simulink model "design_sol"  (R2019b)
settings: Solver=VariableStepAuto  StartTime=0.0  StopTime=10.0  RelTol=1e-3
InitFcn:
  | SSR=8;
undefined symbols (not defined in the file): xc7k325tffg900
libraries: ModelComposer x7, design_lib x2
settings Model: Creator=admin  LastModifiedBy=viswanad
settings DataIOCC: ReturnWorkspaceOutputs=off
settings OptimizationCC: LifeSpan=inf
settings DebuggingCC: ArithmeticOperatorsInVariantConditions=warning
settings SFSimCC: SimUseLocalCustomCode=off  CustomCodeUndefinedFunction=UseInterfaceOnly
settings RTWCC: RTWUseLocalCustomCode=off
settings CodeAppCC: StateflowObjectComments=on

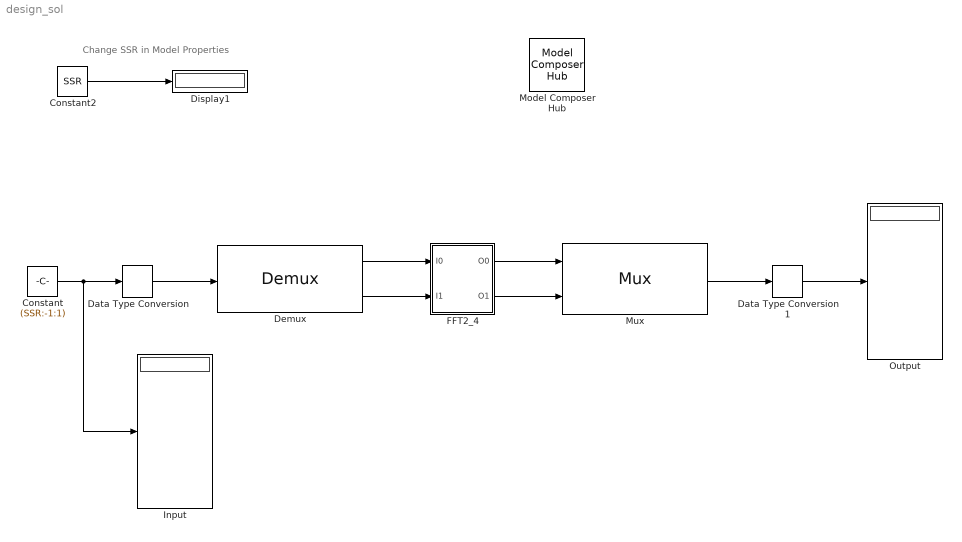
== system design_sol ==
  note: Change SSR in Model Properties
  Constant : Constant  Value=(SSR:-1:1)  SampleTime=1
  Constant2 : Constant  Value=SSR  VectorParams1D=off  SampleTime=1
  Data Type Conversion : ModelComposer/Data Type Conversion  OutDataType=fixed  TypeExp=''  Signedness=Signed  WordLength=16  FractionalLength=8  RoundingMode=Truncation to minus infinity  OverflowMode=Wrap around
  Data Type Conversion1 : ModelComposer/Data Type Conversion  OutDataType=double  TypeExp=''  Signedness=Signed  WordLength=16  FractionalLength=0  RoundingMode=Truncation to minus infinity  OverflowMode=Wrap around
  Demux : design_lib/Demux  LibraryFunction=Demux  IncludeFiles={'template_design.h'}  SourceFiles={}  IncludeDirectories={}  TemplateParams={'int NUMOFELEMENTS'; 'int W'; 'int I'}  FunctionParamTypes={xmcDataType('void'); xmcDataType('ap_fixed<W, I>'); xmcDataType('ap_fixed<W, I>'); xmcDataType('ap_fixed<W, I>')}  FunctionParamPassbys={0.000000000000000000e+00; 0.000000000000000000e+00; 0.000000000000000000e+00; 0.000000000000000000e+00}  FunctionParamDimensions={'1'; '[NUMOFELEMENTS]'; '[NUMOFELEMENTS / 2]'; '[NUMOFELEMENTS / 2]'}  FunctionParamNames={'return'; 'vector_in'; 'vector_out0'; 'vector_out1'}  FunctionParamDir={0.000000000000000000e+00; 1.000000000000000000e+00; 2.000000000000000000e+00; 2.000000000000000000e+00}  FunctionParamSupportsStreaming={false; false; false; false}  BufferDepth={'0'}  FunctionParamValues={'0'; '0'; '0'; '0'}  ThroughputFactors={''}
  Display1 : Display
  FFT2_4 : Subsystem
  Input : Display
  Model Composer Hub : ModelComposer/Model Composer Hub  CodeGeneration=off  SubsystemName=Subsystem  TargetDirectory=./code  ExportType=IP Catalog  IpVendor=xilinx.com  IpLibrary=hls  IpVersion=1.0  IpHWLanguage=Verilog  AieCompilerOptions={}  CreateTestbench=off  TestbenchStackSize=10  RunAieSim=off  AieSimTimeout=50000  LaunchVitisAnalyzer=off  RunX86Sim=on  X86SimTimeout=10  ProjDevice=Kintex-7 KC705 Evaluation Platform (xc7k325tffg900-2)  ProjDevicePart=xc7k325tffg900-2  SamplePeriod=-1  ClockFrequency=200  DataPathParallelism=1
  Mux : design_lib/Mux  LibraryFunction=Mux  IncludeFiles={'template_design.h'}  SourceFiles={}  IncludeDirectories={}  TemplateParams={'int NUMOFELEMENTS'; 'int W'; 'int I'}  FunctionParamTypes={xmcDataType('void'); xmcDataType('ap_fixed<W, I>'); xmcDataType('ap_fixed<W, I>'); xmcDataType('ap_fixed<W, I>')}  FunctionParamPassbys={0.000000000000000000e+00; 0.000000000000000000e+00; 0.000000000000000000e+00; 0.000000000000000000e+00}  FunctionParamDimensions={'1'; '[NUMOFELEMENTS]'; '[NUMOFELEMENTS]'; '[NUMOFELEMENTS * 2]'}  FunctionParamNames={'return'; 'vector_in0'; 'vector_in1'; 'vector_out'}  FunctionParamDir={0.000000000000000000e+00; 1.000000000000000000e+00; 1.000000000000000000e+00; 2.000000000000000000e+00}  FunctionParamSupportsStreaming={false; false; false; false}  BufferDepth={'0'}  FunctionParamValues={'0'; '0'; '0'; '0'}  ThroughputFactors={''}
  Output : Display
  wires:
  Constant/1 -> Input/1, Data Type Conversion/1
  Data Type Conversion1/1 -> Output/1
  Data Type Conversion/1 -> Demux/1
  Mux/1 -> Data Type Conversion1/1
  FFT2_4/1(O0) -> Mux/1
  FFT2_4/2(O1) -> Mux/2
  Demux/1 -> FFT2_4/1(I0)
  Demux/2 -> FFT2_4/2(I1)
  Constant2/1 -> Display1/1

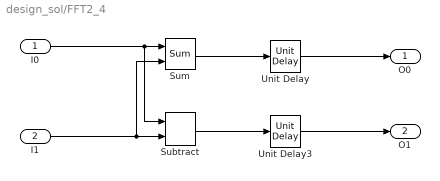
== system design_sol/FFT2_4 ==
  I0 : Inport
  I1 : Inport  Port=2
  Subtract : ModelComposer/Subtract
  Sum : ModelComposer/Sum
  Unit Delay : ModelComposer/Unit Delay  InitialCondition=0
  Unit Delay3 : ModelComposer/Unit Delay  InitialCondition=0
  O0 : Outport
  O1 : Outport  Port=2
  wires:
  Sum/1 -> Unit Delay/1
  Unit Delay/1 -> O0/1
  Subtract/1 -> Unit Delay3/1
  Unit Delay3/1 -> O1/1
  I0/1 -> Subtract/1, Sum/1
  I1/1 -> Subtract/2, Sum/2
